simulink model "sampleModel1724"  (R2023a)
settings: Solver=VariableStepAuto  StartTime=0.0  StopTime=10.0  RelTol=1e-3
libraries: hdlsllib x5, simulink x2
settings Model: Creator=user1  LastModifiedBy=user1

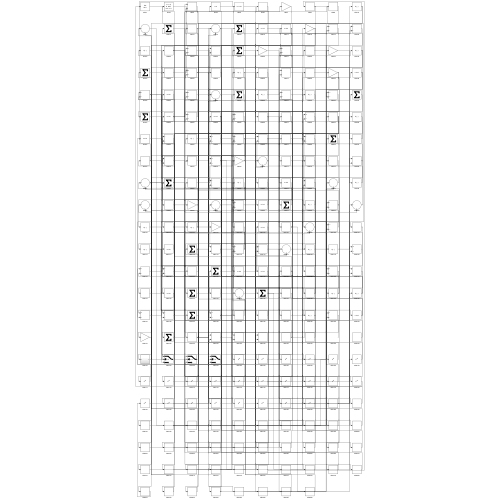
[thumbnail: Simulink's stored preview of the top-level diagram]
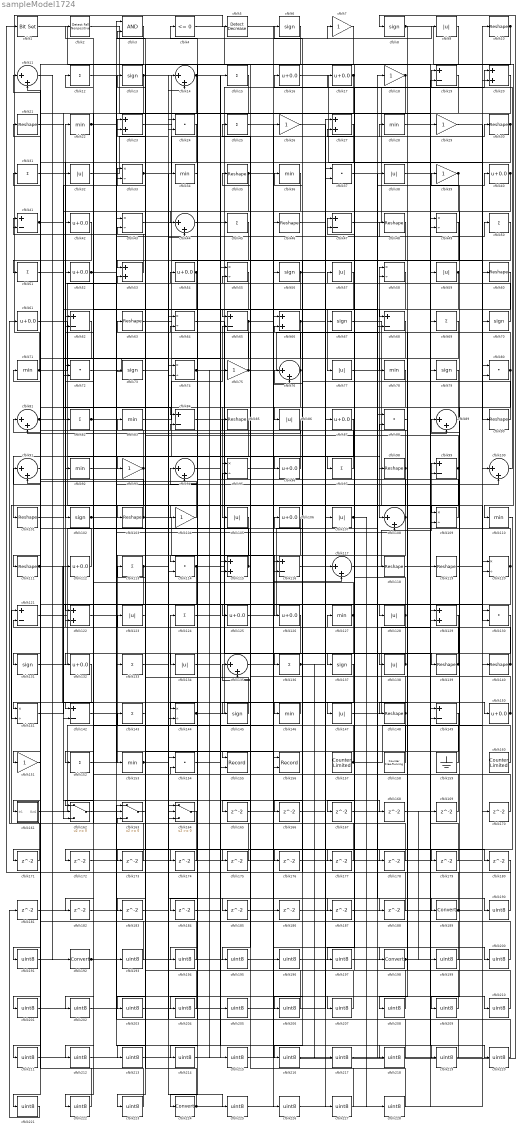
== system sampleModel1724 ==
  cfblk1 : simulink/Logic and Bit Operations/Bit Set  iBit=0
      settings: LibrarySourceBlock=|
      | hdlsllib/Logic and Bit
      | Operations/Bit Set
  cfblk{10,21,30,35,46,48,60,63,85,90,98,101,103,111,118..119,139..140,148} (19 alike) : Reshape
  cfblk{11,14,44,76,81,89,91,94,100,108,117,135} (12 alike) : Sum  Inputs=|++
  cfblk{6,8,13,56,67,70,73,79,102,131,137,145} (12 alike) : Signum
  cfblk{7,18,26,29,39,75,93,104,151} (9 alike) : Gain
  cfblk{9,32,38,57,59,77,86,105,107,123,128,134,138,147} (14 alike) : Abs  SaturateOnIntegerOverflow=off
  cfblk{16..17,40,42,52,54,61,87,96,106,112,125..126,132,150} (15 alike) : Bias  Bias=0.0  SaturateOnIntegerOverflow=off
  cfblk{33,43,49,55,58,64,74,95,109,120,141,144} (12 alike) : Product  Inputs=*/  RndMeth=Zero  SaturateOnIntegerOverflow=on
  cfblk{22,28,34,36,71,78,83,92,110,127,146,153} (12 alike) : MinMax
  cfblk{12,15,25,31,45,50..51,69,82,97,113,124,133,136,143,152} (16 alike) : Sum  Inputs=+
  cfblk{24,37,72,80,88,114,130,154} (8 alike) : DotProduct  OutDataTypeStr=Inherit: Inherit via internal rule
  cfblk{20,23,27,53,66,115,122,129} (8 alike) : Sum
  cfblk{19,41,47,62,65,68,84,99,116,121,142,149} (12 alike) : Sum  Inputs=+-
  cfblk155 : Record  FileSettingsInternal="{\"entries\":[{\"content\":{\"excelSettings\":{\"content\":{},\"type\":\"Streamout.ExcelSettings\"}},\"type\":\"Streamout.FileSettingStorage\",\"uuid\":\"\"}],\"packageUris\":[\"http:\\/\\/schema.mathworks.com\\/mf0\\/streamout_blocks\\/R2020a\"],\"version\":\"1.0\"}"  Layout=[1 1]  SignalsInternal="{\"entries\":[{\"content\":{\"signals\":[{\"content\":{\"blockPath\":[],\"dimensions\":[1],\"domain\":\"\",\"lineColor\":\"#a2142f\",\"plots\":[1],\"port\":1,\"signalID\":3329,\"signalName\":\"XY Graph:1\"},\"type\":\"RecordBlkView.Signal\",\"uuid\":\"\"},{\"content\":{\"blockPath\":[],\"dimensions\":[1],\"domain\":\"\",\"lineColor\":\"#139fff\",\"plots\":[1],\"port\":2,\"signalID\":3332,\"signalName\":\"XY Graph:2\"},\"type\":\"RecordBlkView.Signal\",\"uuid\":\"\"}]},\"type\":\"RecordBlkView.InputSignals\",\"uuid\":\"\"}],\"packageUris\":[\"http:\\/\\/schema.mathworks.com\\/mf0\\/streamout_blocks\\/R2020a\"],\"version\":\"1.0\"}"  VisualizationBindings="{\"xyplotplugin\":{\"info\":[{\"series\":[{\"bindingParametersList\":[{\"parameter\":\"X-Axis\",\"signalID\":3329,\"signalName\":\"XY Graph:1\"},{\"parameter\":\"Y-Axis\",\"signalID\":3332,\"signalName\":\"XY Graph:2\"}],\"seriesID\":6063}],\"subplotID\":1}]}}"  CompatibilityTag=XY  st=-1
  cfblk156 : Record  FileSettingsInternal="{\"entries\":[{\"content\":{\"excelSettings\":{\"content\":{},\"type\":\"Streamout.ExcelSettings\"}},\"type\":\"Streamout.FileSettingStorage\",\"uuid\":\"\"}],\"packageUris\":[\"http:\\/\\/schema.mathworks.com\\/mf0\\/streamout_blocks\\/R2020a\"],\"version\":\"1.0\"}"  Layout=[1 1]  SignalsInternal="{\"entries\":[{\"content\":{\"signals\":[{\"content\":{\"blockPath\":[],\"dimensions\":[1],\"domain\":\"\",\"lineColor\":\"#a2142f\",\"plots\":[1],\"port\":1,\"signalID\":3337,\"signalName\":\"XY Graph:1\"},\"type\":\"RecordBlkView.Signal\",\"uuid\":\"\"},{\"content\":{\"blockPath\":[],\"dimensions\":[1],\"domain\":\"\",\"lineColor\":\"#139fff\",\"plots\":[1],\"port\":2,\"signalID\":3340,\"signalName\":\"XY Graph:2\"},\"type\":\"RecordBlkView.Signal\",\"uuid\":\"\"}]},\"type\":\"RecordBlkView.InputSignals\",\"uuid\":\"\"}],\"packageUris\":[\"http:\\/\\/schema.mathworks.com\\/mf0\\/streamout_blocks\\/R2020a\"],\"version\":\"1.0\"}"  VisualizationBindings="{\"xyplotplugin\":{\"info\":[{\"series\":[{\"bindingParametersList\":[{\"parameter\":\"X-Axis\",\"signalID\":3337,\"signalName\":\"XY Graph:1\"},{\"parameter\":\"Y-Axis\",\"signalID\":3340,\"signalName\":\"XY Graph:2\"}],\"seriesID\":57072}],\"subplotID\":1}]}}"  CompatibilityTag=XY  st=-1
  cfblk157 : hdlsllib/Sources/Counter Limited  uplimit=7  tsamp=-1
  cfblk158 : hdlsllib/Sources/Counter Free-Running  NumBits=16  tsamp=-1
  cfblk159 : Ground
  cfblk160 : hdlsllib/Sources/Counter Limited  uplimit=7  tsamp=-1
  cfblk161 : Subsystem
      settings: LibrarySourceBlock=|
      | hdlsllib/Ports &
      | Subsystems/Subsystem
  cfblk162 : Switch  SaturateOnIntegerOverflow=off  InputSameDT=off
  cfblk163 : Switch  SaturateOnIntegerOverflow=off  InputSameDT=off
  cfblk164 : Switch  SaturateOnIntegerOverflow=off  InputSameDT=off
  cfblk{165..188} (24 alike) : Delay  SampleTime=1
  cfblk{189,192,198,224} (4 alike) : DataTypeConversion  SaturateOnIntegerOverflow=off  RndMeth=Floor
  cfblk{190..191,193..197,199..223,225..228} (36 alike) : DataTypeConversion  OutDataTypeStr=uint8  SaturateOnIntegerOverflow=off  RndMeth=Floor
  cfblk2 : hdlsllib/Logic and Bit Operations/Detect Fall Nonpositive  vinit=0  OutDataTypeStr=boolean
  cfblk3 : Logic  AllPortsSameDT=off  OutDataTypeStr=boolean
  cfblk4 : hdlsllib/Logic and Bit Operations/Compare To Zero  relop=<=  OutDataTypeStr=boolean
  cfblk5 : simulink/Logic and Bit Operations/Detect Decrease  vinit=0.0  OutDataTypeStr=boolean
      settings: LibrarySourceBlock=|
      | hdlsllib/Logic and Bit
      | Operations/Detect
      | Decrease
  wires:
  cfblk140/1 -> cfblk22/1, cfblk63/1
  cfblk129/1 -> cfblk136/1
  cfblk54/1 -> cfblk212/1, cfblk214/1
  cfblk114/1 -> cfblk137/1, cfblk202/1
  cfblk57/1 -> cfblk77/1
  cfblk40/1 -> cfblk73/1, cfblk68/1
  cfblk13/1 -> cfblk108/1, cfblk51/1
  cfblk100/1 -> cfblk16/1
  cfblk111/1 -> cfblk147/1, cfblk130/2
  cfblk105/1 -> cfblk153/1
  cfblk47/1 -> cfblk20/1
  cfblk49/1 -> cfblk53/1
  cfblk150/1 -> cfblk57/1, cfblk95/2
  cfblk159/1 -> cfblk124/1
  cfblk85/1 -> cfblk101/1
  cfblk69/1 -> cfblk224/1
  cfblk117/1 -> cfblk99/1
  cfblk115/1 -> cfblk54/1, cfblk82/1
  cfblk19/1 -> cfblk49/2
  cfblk37/1 -> cfblk189/1
  cfblk59/1 -> cfblk97/1, cfblk152/1, cfblk114/2, cfblk165/1
  cfblk102/1 -> cfblk156/2, cfblk222/1
  cfblk8/1 -> cfblk110/1, cfblk148/1
  cfblk90/1 -> cfblk36/1
  cfblk144/1 -> cfblk19/1, cfblk180/1
  cfblk31/1 -> cfblk102/1
  cfblk6/1 -> cfblk133/1
  cfblk89/1 -> cfblk86/1
  cfblk74/1 -> cfblk139/1, cfblk215/1
  cfblk99/1 -> cfblk128/1, cfblk33/1
  cfblk9/1 -> cfblk93/1
  cfblk30/1 -> cfblk103/1, cfblk184/1
  cfblk52/1 -> cfblk50/1, cfblk7/1
  cfblk23/1 -> cfblk80/2
  cfblk133/1 -> cfblk64/1
  cfblk42/1 -> cfblk141/1
  cfblk119/1 -> cfblk10/1
  cfblk163/1 -> cfblk23/1
  cfblk2/1 -> cfblk119/1
  cfblk60/1 -> cfblk65/1
  cfblk158/1 -> cfblk6/1
  cfblk131/1 -> cfblk46/1
  cfblk121/1 -> cfblk24/2
  cfblk123/1 -> cfblk13/1
  cfblk128/1 -> cfblk121/2, cfblk85/1
  cfblk112/1 -> cfblk81/1
  cfblk101/1 -> cfblk146/1
  cfblk27/1 -> cfblk151/1
  cfblk18/1 -> cfblk144/1, cfblk104/1
  cfblk43/1 -> cfblk87/1
  cfblk35/1 -> cfblk117/2, cfblk142/2
  cfblk11/1 -> cfblk192/1
  cfblk138/1 -> cfblk52/1, cfblk84/2
  cfblk76/1 -> cfblk105/1, cfblk4/1
  cfblk4/1 -> cfblk56/1
  cfblk80/1 -> cfblk35/1, cfblk209/1
  cfblk71/1 -> cfblk5/1, cfblk43/1
  cfblk145/1 -> cfblk123/1
  cfblk104/1 -> cfblk31/1
  cfblk139/1 -> cfblk127/1, cfblk39/1
  cfblk29/1 -> cfblk90/1
  cfblk127/1 -> cfblk62/1, cfblk162/1, cfblk167/1
  cfblk56/1 -> cfblk132/1, cfblk188/1
  cfblk164/1 -> cfblk61/1
  cfblk93/1 -> cfblk21/1, cfblk141/2
  cfblk75/1 -> cfblk58/1, cfblk43/2
  cfblk14/1 -> cfblk115/1, cfblk162/2
  cfblk39/1 -> cfblk155/1, cfblk129/2
  cfblk16/1 -> cfblk70/1
  cfblk67/1 -> cfblk130/1
  cfblk98/1 -> cfblk47/1, cfblk2/1, cfblk162/3
  cfblk61/1 -> cfblk118/1
  cfblk38/1 -> cfblk19/2
  cfblk51/1 -> cfblk67/1
  cfblk63/1 -> cfblk155/2
  cfblk86/1 -> cfblk81/2
  cfblk152/1 -> cfblk108/2
  cfblk113/1 -> cfblk122/1, cfblk187/1
  cfblk3/1 -> cfblk161/1(In1)
  cfblk24/1 -> cfblk32/1
  cfblk65/1 -> cfblk144/2, cfblk138/1
  cfblk81/1 -> cfblk96/1, cfblk33/2
  cfblk66/1 -> cfblk107/1, cfblk111/1
  cfblk120/1 -> cfblk66/2, cfblk201/1
  cfblk134/1 -> cfblk45/1
  cfblk33/1 -> cfblk30/1, cfblk185/1
  cfblk64/1 -> cfblk109/1
  cfblk153/1 -> cfblk48/1, cfblk44/2, cfblk225/1
  cfblk41/1 -> cfblk84/1, cfblk168/1
  cfblk141/1 -> cfblk112/1
  cfblk160/1 -> cfblk89/1
  cfblk82/1 -> cfblk12/1, cfblk210/1
  cfblk36/1 -> cfblk164/3
  cfblk103/1 -> cfblk71/1, cfblk126/1
  cfblk83/1 -> cfblk65/2
  cfblk68/1 -> cfblk98/1
  cfblk53/1 -> cfblk41/1
  cfblk107/1 -> cfblk47/2, cfblk228/1
  cfblk84/1 -> cfblk129/1
  cfblk70/1 -> cfblk42/1
  cfblk34/1 -> cfblk114/1
  cfblk125/1 -> cfblk40/1
  cfblk146/1 -> cfblk145/1
  cfblk157/1 -> cfblk60/1, cfblk72/1
  cfblk1/1 -> cfblk79/1
  cfblk96/1 -> cfblk83/1
  cfblk21/1 -> cfblk74/2
  cfblk17/1 -> cfblk142/1, cfblk72/2
  cfblk108/1 -> cfblk125/1, cfblk53/2
  cfblk147/1 -> cfblk89/2
  cfblk62/1 -> cfblk92/1
  cfblk32/1 -> cfblk14/2
  cfblk124/1 -> cfblk75/1
  cfblk161/1(Out1) -> cfblk26/1
  cfblk92/1 -> cfblk100/2
  cfblk46/1 -> cfblk28/1
  cfblk10/1 -> cfblk44/1, cfblk177/1
  cfblk79/1 -> cfblk131/1
  cfblk136/1 -> cfblk150/1, cfblk217/1
  cfblk142/1 -> cfblk3/1
  cfblk25/1 -> cfblk198/1
  cfblk109/1 -> cfblk76/1
  cfblk122/1 -> cfblk9/1
  cfblk7/1 -> cfblk95/1
  cfblk20/1 -> cfblk134/1
  cfblk22/1 -> cfblk68/2, cfblk175/1
  cfblk73/1 -> cfblk34/1
  cfblk77/1 -> cfblk58/2
  cfblk148/1 -> cfblk17/1, cfblk173/1
  cfblk97/1 -> cfblk64/2
  cfblk165/1 -> cfblk66/1
  cfblk48/1 -> cfblk166/1
  cfblk166/1 -> cfblk117/1
  cfblk167/1 -> cfblk99/2
  cfblk168/1 -> cfblk109/2
  cfblk169/1 -> cfblk23/2
  cfblk170/1 -> cfblk62/2
  cfblk151/1 -> cfblk171/1
  cfblk171/1 -> cfblk121/1
  cfblk110/1 -> cfblk172/1
  cfblk172/1 -> cfblk100/1
  cfblk173/1 -> cfblk41/2
  cfblk106/1 -> cfblk174/1
  cfblk174/1 -> cfblk24/1
  cfblk175/1 -> cfblk3/2
  cfblk44/1 -> cfblk176/1
  cfblk177/1 -> cfblk163/3
  cfblk162/1 -> cfblk178/1
  cfblk178/1 -> cfblk122/2
  cfblk72/1 -> cfblk179/1
  cfblk179/1 -> cfblk49/1
  cfblk180/1 -> cfblk1/1
  cfblk181/1 -> cfblk74/1
  cfblk87/1 -> cfblk182/1
  cfblk126/1 -> cfblk183/1
  cfblk183/1 -> cfblk14/1
  cfblk184/1 -> cfblk115/2
  cfblk185/1 -> cfblk76/2
  cfblk186/1 -> cfblk80/1
  cfblk187/1 -> cfblk120/2
  cfblk188/1 -> cfblk163/1
  cfblk189/1 -> cfblk140/1, cfblk106/1
  cfblk26/1 -> cfblk190/1
  cfblk190/1 -> cfblk37/1
  cfblk132/1 -> cfblk191/1
  cfblk191/1 -> cfblk37/2
  cfblk192/1 -> cfblk38/1, cfblk156/1, cfblk18/1
  cfblk12/1 -> cfblk193/1
  cfblk193/1 -> cfblk11/1
  cfblk130/1 -> cfblk194/1
  cfblk194/1 -> cfblk11/2
  cfblk149/1 -> cfblk195/1
  cfblk195/1 -> cfblk29/1
  cfblk5/1 -> cfblk196/1
  cfblk196/1 -> cfblk149/1
  cfblk58/1 -> cfblk197/1
  cfblk197/1 -> cfblk149/2
  cfblk198/1 -> cfblk170/1, cfblk169/1
  cfblk118/1 -> cfblk199/1
  cfblk199/1 -> cfblk25/1
  cfblk116/1 -> cfblk200/1
  cfblk200/1 -> cfblk164/1
  cfblk201/1 -> cfblk116/1
  cfblk202/1 -> cfblk116/2
  cfblk143/1 -> cfblk203/1
  cfblk203/1 -> cfblk164/2
  cfblk45/1 -> cfblk204/1
  cfblk204/1 -> cfblk143/1
  cfblk94/1 -> cfblk205/1
  cfblk205/1 -> cfblk27/1
  cfblk137/1 -> cfblk206/1
  cfblk206/1 -> cfblk94/1
  cfblk95/1 -> cfblk207/1
  cfblk207/1 -> cfblk94/2
  cfblk88/1 -> cfblk208/1
  cfblk208/1 -> cfblk27/2
  cfblk209/1 -> cfblk88/1
  cfblk210/1 -> cfblk88/2
  cfblk15/1 -> cfblk211/1
  cfblk211/1 -> cfblk120/1
  cfblk212/1 -> cfblk15/1
  cfblk55/1 -> cfblk213/1
  cfblk213/1 -> cfblk186/1
  cfblk214/1 -> cfblk55/1
  cfblk215/1 -> cfblk55/2
  cfblk78/1 -> cfblk216/1
  cfblk216/1 -> cfblk8/1
  cfblk217/1 -> cfblk78/1
  cfblk154/1 -> cfblk218/1
  cfblk218/1 -> cfblk163/2
  cfblk182/1 -> cfblk219/1
  cfblk219/1 -> cfblk154/1
  cfblk28/1 -> cfblk220/1
  cfblk220/1 -> cfblk154/2
  cfblk91/1 -> cfblk221/1
  cfblk221/1 -> cfblk181/1
  cfblk222/1 -> cfblk91/1
  cfblk50/1 -> cfblk223/1
  cfblk223/1 -> cfblk91/2
  cfblk224/1 -> cfblk20/2, cfblk113/1
  cfblk225/1 -> cfblk69/1
  cfblk135/1 -> cfblk226/1
  cfblk226/1 -> cfblk59/1
  cfblk176/1 -> cfblk227/1
  cfblk227/1 -> cfblk135/1
  cfblk228/1 -> cfblk135/2

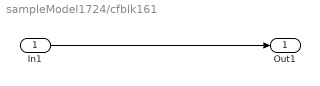
== system sampleModel1724/cfblk161 ==
  In1 : Inport
  Out1 : Outport
  wires:
  In1/1 -> Out1/1
